simulink model "modellutenkobling"  (R2025b)
settings: Solver=ode1  StartTime=0.0  StopTime=3  FixedStep=1e-3  MaxStep=10e-9  RelTol=1e-9
values from neighbouring files (symbols this model uses):
  avstand_t0 = 400    [data 2.m]    (also in data.m = 0)
  K = 0.89    [data 2.m]    (also in data.m = 0.96)
  kb = 4    [data.m]
  Kd = Kp*Td    (= 0)    [data 2.m]    (also in data.m)
  Ki = 0    [data 2.m]    (also in data.m)
  Kp = 4    [data 2.m]    (also in data.m = 5.21)
  setpoint = 200    [data 2.m]    (also in data.m = 100)
  Tau = 0.04    [data 2.m]    (also in data.m = 0.1)
settings Model: Creator=akselludvigsenholmas  LastModifiedBy=alexa

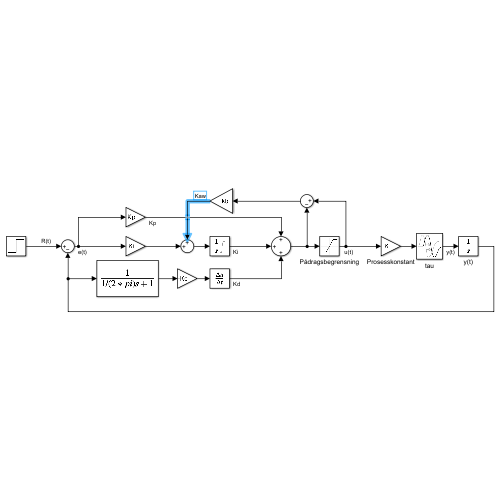
[thumbnail: Simulink's stored preview of the top-level diagram]
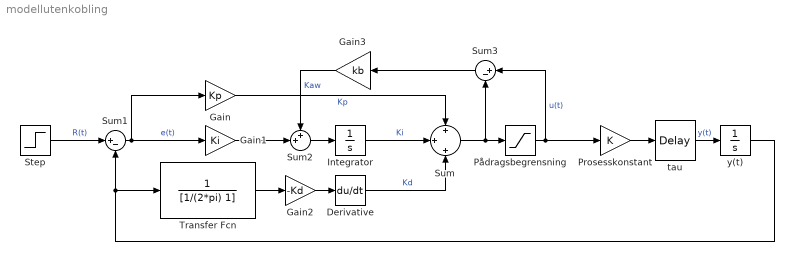
== system modellutenkobling ==
  Derivative : Derivative
  Gain : Gain  Gain=Kp
  Gain1 : Gain  Gain=Ki
  Gain2 : Gain  Gain=-Kd
  Gain3 : Gain  Gain=kb
  Integrator : Integrator  LimitOutput=on  UpperSaturationLimit=250  LowerSaturationLimit=-250
  Prosesskonstant : Gain  Gain=K
  Pådragsbegrensning : Saturate  UpperLimit=250  LowerLimit=-250
  Step : Step  Time=0.1  After=setpoint  SampleTime=0
  Sum : Sum  Inputs=+|+|+
  Sum1 : Sum  Inputs=|+-
  Sum2 : Sum  Inputs=++|
  Sum3 : Sum  Inputs=|+-
  Transfer Fcn : TransferFcn  Denominator=[1/(2*pi) 1]
  tau : TransportDelay  DelayTime=Tau  InitialOutput=avstand_t0  BufferSize=2^16
  y(t) : Integrator  InitialCondition=avstand_t0
  wires:
  Step/1 -> Sum1/1  "R(t)"
  Pådragsbegrensning/1 -> Prosesskonstant/1, Sum3/1  "u(t)"
  Sum/1 -> Sum3/2, Pådragsbegrensning/1
  Gain2/1 -> Derivative/1
  Derivative/1 -> Sum/3  "Kd"
  Transfer Fcn/1 -> Gain2/1
  tau/1 -> y(t)/1  "y(t)"
  Gain/1 -> Sum/1  "Kp"
  Prosesskonstant/1 -> tau/1
  y(t)/1 -> Sum1/2, Transfer Fcn/1
  Integrator/1 -> Sum/2  "Ki"
  Sum1/1 -> Gain1/1, Gain/1  "e(t)"
  Sum2/1 -> Integrator/1
  Gain1/1 -> Sum2/2
  Sum3/1 -> Gain3/1
  Gain3/1 -> Sum2/1  "Kaw"
